simulink model "linear_ode_model"  (R2024a)
settings: Solver=ode45  StartTime=0  StopTime=5  MaxStep=0.01  RelTol=1e-3
settings Model: Creator=andrey  LastModifiedBy=andrey

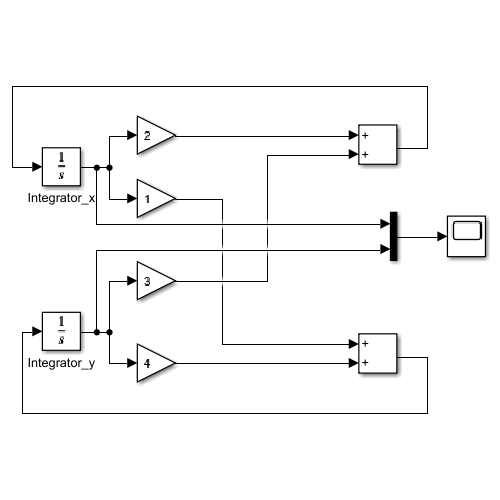
[thumbnail: Simulink's stored preview of the top-level diagram]
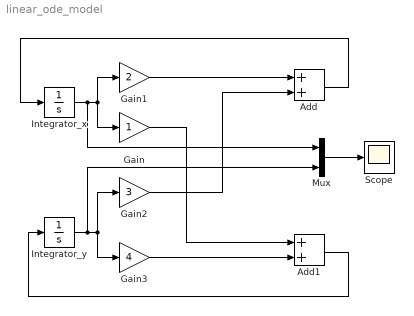
== system linear_ode_model ==
  Add : Sum
  Add1 : Sum
  Gain : Gain
  Gain1 : Gain  Gain=2
  Gain2 : Gain  Gain=3
  Gain3 : Gain  Gain=4
  Integrator_x : Integrator  InitialCondition=1
  Integrator_y : Integrator
  Mux : Mux  Inputs=2
  Scope : Scope
  wires:
  Integrator_x/1 -> Mux/1, Gain/1, Gain1/1
  Integrator_y/1 -> Mux/2, Gain3/1, Gain2/1
  Gain1/1 -> Add/1
  Gain2/1 -> Add/2
  Add/1 -> Integrator_x/1
  Gain/1 -> Add1/1
  Gain3/1 -> Add1/2
  Add1/1 -> Integrator_y/1
  Mux/1 -> Scope/1
